simulink model "imp"  (R2019b)
settings: Solver=VariableStepAuto  StartTime=0.0  StopTime=25  MaxStep=0.01  RelTol=1e-3
undefined symbols (not defined in the file): c, k, m, sigbuilder_block
libraries: simulink x1, simulink_extras x1
settings Model: Creator=EREN  LastModifiedBy=EREN

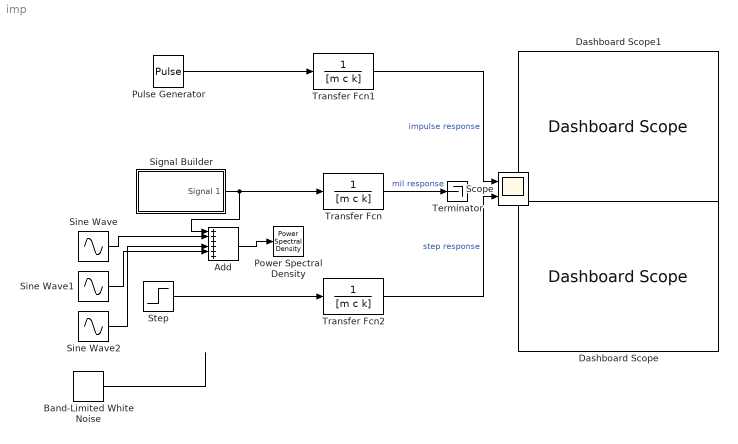
== system imp ==
  Add : Sum  Inputs=++++++
  Band-Limited White Noise : simulink/Sources/Band-Limited White Noise  Cov=1  Ts=1/20  seed=[23341]
  Dashboard Scope : DashboardScope  Ymin=0  Ymax=5
  Dashboard Scope1 : DashboardScope  Ymin=0  Ymax=5
  Power Spectral Density : simulink_extras/Additional Sinks/Power Spectral Density  npts=128  fftpts=512  HowOften=64  sampleT=0.01
      settings: SourceProductName=Simulink  SourceProductBaseCode=SL
  Pulse Generator : DiscretePulseGenerator  PulseType=Time based  Amplitude=20*9.8  Period=100  PulseWidth=0.01
  Scope : Scope  NumInputPorts=2
  Signal Builder : Subsystem  Tag=STV Subsys  LoadFcn=sigbuilder_block('load');  StartFcn=sigbuilder_block('start');  StopFcn=sigbuilder_block('stop');  ClipboardFcn=sigbuilder_block('clipboard');  mask(Sigbuilder block){tuvar=[0:10]}
      mask help: Simulink:masks:SigbuilderBlock_MD
      mask init:
      | if ~strcmp(get_param(bdroot(gcbh),'SimulationStatus'),'stopped') tuvar = sigbuilder_block('maskInit'); end
      settings: CopyFcn=sigbuilder_block('copy');  DeleteFcn=sigbuilder_block('delete');  ModelCloseFcn=sigbuilder_block('modelClose');  PreSaveFcn=sigbuilder_block('preSave');  PauseFcn=sigbuilder_block('pause');  ContinueFcn=sigbuilder_block('continue');  NameChangeFcn=sigbuilder_block('namechange');  OpenFcn=sigbuilder_block('open',[225.6 120 550.8 400.2 ]);  CloseFcn=sigbuilder_block('close');
      mask Display: plot(0, 0, 100, 100,[2, 2, 32, 32, 2], [68, 8, 8, 68, 68],[32, 2], [38, 38], [32, 19, 2],[53, 60, 44], [32, 17, 17, 2],[16, 16, 31, 31]);txt = getActiveGroup(gcbh);text(2, 100, txt,'verticalAlignment', 'top');
  Sine Wave : Sin  Frequency=300  SampleTime=0
  Sine Wave1 : Sin  Frequency=20  SampleTime=0
  Sine Wave2 : Sin  Frequency=200  SampleTime=0
  Step : Step  Time=0  After=2  SampleTime=0
  Terminator : Terminator
  Transfer Fcn : TransferFcn  Denominator=[m c k]
  Transfer Fcn1 : TransferFcn  Denominator=[m c k]
  Transfer Fcn2 : TransferFcn  Denominator=[m c k]
  wires:
  Transfer Fcn/1 -> Terminator/1  "mil response"
  Signal Builder/1(Signal 1) -> Add/1, Transfer Fcn/1
  Pulse Generator/1 -> Transfer Fcn1/1
  Transfer Fcn1/1 -> Scope/1  "impulse response"
  Step/1 -> Transfer Fcn2/1
  Transfer Fcn2/1 -> Scope/2  "step response"
  Sine Wave/1 -> Add/2
  Add/1 -> Power Spectral Density/1
  Sine Wave1/1 -> Add/5
  Sine Wave2/1 -> Add/4
  Band-Limited White Noise/1 -> ?

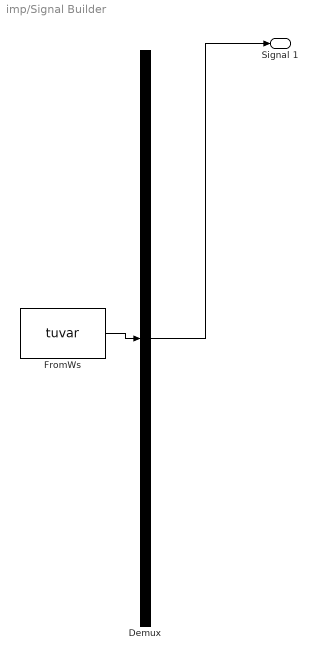
== system imp/Signal Builder ==
  Demux : Demux  Tag=STV Demux  Outputs=1
  FromWs : FromWorkspace  Tag=STV FromWs  VariableName=tuvar  SampleTime=0
      SigBuilderData=|
      | common.afterFinalStr = 'Extrapolate'
      | common.sampleTime = 0
      | dataSet.timeRange = [0 10]
      | dataSet.name = 'Group 1'
      | sbobj.Groups.Name = 'Group 1'
      | sbobj.Groups.Signals.Name = 'Signal 1'
      | sbobj.Groups.Signals.XData = [0 4 6 6 10]
      | sbobj.Groups.Signals.YData = [0 197 196 3 0]
  Signal 1 : Outport  Tag=STV Outport
  wires:
  Demux/1 -> Signal 1/1
  FromWs/1 -> Demux/1
